simulink subsystem "s1EM"  (R2023b)
settings: Solver=VariableStepAuto  StartTime=0.0  StopTime=10.0  RelTol=1e-3
settings Model: Creator=The MathWorks, Inc.  LastModifiedBy=The MathWorks, Inc.

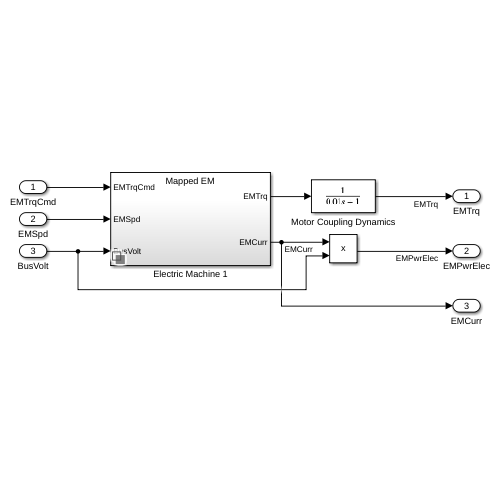
[thumbnail: Simulink's stored preview of the top-level diagram]
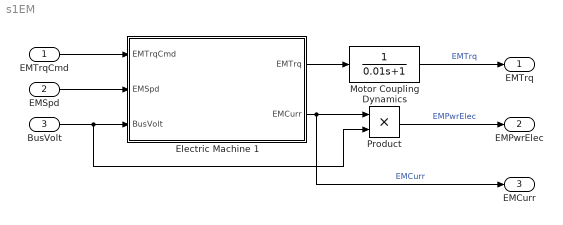
== system s1EM ==
  EMTrqCmd : Inport
  EMSpd : Inport  Port=2
  BusVolt : Inport  Port=3
  Electric Machine 1 : Subsystem  Variant=on  VariantControlMode=label  LabelModeActiveChoice=Mapped EM
  Motor Coupling Dynamics : TransferFcn  Denominator=[0.01 1]
  Product : Product
  EMTrq : Outport
  EMPwrElec : Outport  Port=2
  EMCurr : Outport  Port=3
  wires:
  Motor Coupling Dynamics/1 -> EMTrq/1  "EMTrq"
  EMTrqCmd/1 -> Electric Machine 1/1(EMTrqCmd)
  BusVolt/1 -> Product/2, Electric Machine 1/3(BusVolt)
  Product/1 -> EMPwrElec/1  "EMPwrElec"
  EMSpd/1 -> Electric Machine 1/2(EMSpd)
  Electric Machine 1/2(EMCurr) -> EMCurr/1, Product/1  "EMCurr"
  Electric Machine 1/1(EMTrq) -> Motor Coupling Dynamics/1

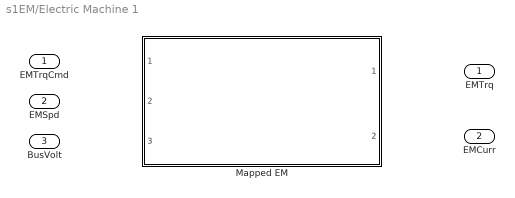
== system s1EM/Electric Machine 1 ==
  EMTrqCmd : Inport
  EMSpd : Inport  Port=2
  BusVolt : Inport  Port=3
  Mapped EM : Subsystem  VariantControl=Mapped EM  ReferencedSubsystem=ElectricMachine1
  EMTrq : Outport  VectorParamsAs1DForOutWhenUnconnected=off
  EMCurr : Outport  Port=2  VectorParamsAs1DForOutWhenUnconnected=off
